simulink model "ErskineMultiDroneFormation_5drones"  (R2019b)
settings: Solver=FixedStepAuto  StartTime=0.0  StopTime=Tsim  FixedStep=sim_dt  RelTol=1e-3
values from neighbouring files (symbols this model uses):
  controller_rate = 50    [MultiQuadInit.m]
  drone_params = setDefaultDroneParams(nDrones)    [MultiQuadInit.m]
  dt_p = 0.2    [MultiQuadInit.m]    (also in setSimConditions.m)
  edges = [1,2 ... (first row only)    [MultiQuadInit.m]    (also in setSimConditions.m)
  g = 9.81    [MultiQuadInit.m]
  N_p = 5    [MultiQuadInit.m]    (also in setSimConditions.m)
  nDrones = 3    [MultiQuadInit.m]
  omega0 = zeros(3,nDrones)    [MultiQuadInit.m]    (also in setSimConditions.m)
  p0 = scale*(rand(3,nDrones) - [0.5;0.5;0])    [MultiQuadInit.m]    (also in setSimConditions.m = scale*(rand(3,nDrones) - [1/2;1/2;0]))
  q0 = zeros(4,nDrones); q0(1,:) = ones(1,nDrones)    [MultiQuadInit.m]    (also in setSimConditions.m)
  sim_dt = 0.005    [MultiQuadInit.m]
  v0 = zeros(3, nDrones)    [MultiQuadInit.m]    (also in setSimConditions.m)
undefined symbols (not defined in the file or in its folder): camera_noise
libraries: vrlib x13
(part 1 of 4)
settings Model: Creator=julian  LastModifiedBy=julian

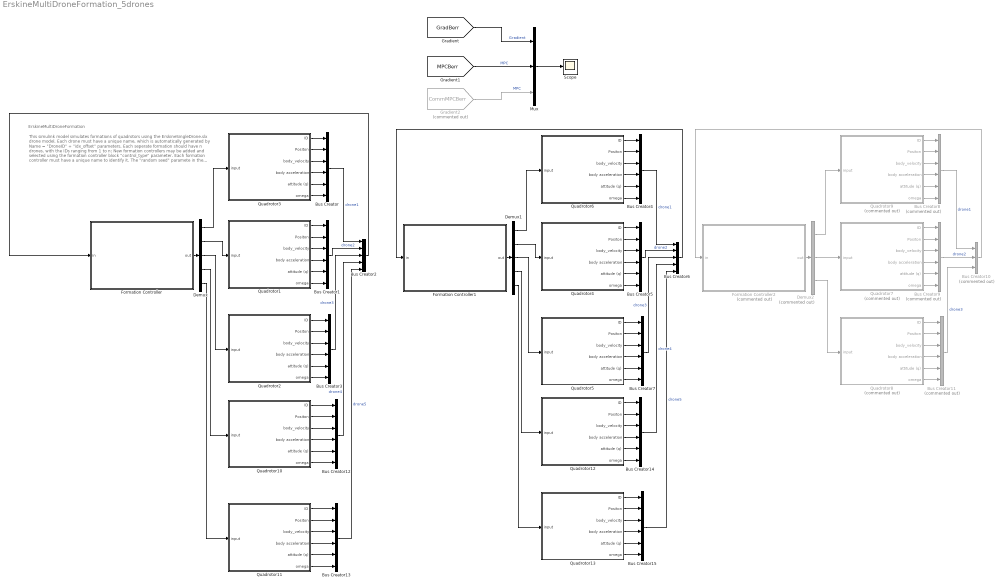
== system ErskineMultiDroneFormation_5drones ==
  note: This simulink model simulates formations of quadrotors using the
      | ErskineSingleDrone.slx drone model.  Each drone must have a unique name,
      | which is automatically generated by Name = "DroneID" + "idx_offset" parameters.
      | Each seperate formation should have n drones, with the IDs ranging from 1 to n;
      |
      | New formation controllers may be added and selected using the formation
      | controller block "control_type" parameter. Each formation controller must have a
      | unique name to identify it. The "random seed" paramete in the formation control block sets the random noise seed for the controller measurements.
      |
      | Initial conditions, parameters, and the FormationStateBus must be generated for n drones (see initialization script)
  note: ErskineMultiDroneFormation
  "  Quadrotor1" : Subsystem  mask{control_type_param=2: Body Velocity + Yawrate, DroneID=2, DroneName=Drone2, idx_offset=0}
      mask prompts: control_type_param "Controller type"; DroneName "Drone Name"; idx_offset "Index Offset"
      mask TypeOptions control_type_param: 1: Position + Yaw | 2: Body Velocity + Yawrate | 3: Body Acceleration + Yawrate | 4: Thrust + Attitude | 5: Thrust + Body Rate | 6: Body Wrench
      mask TypeOptions DroneID: 1 | 2 | 3 | 4 | 5 | 6 | 7 | 8 | 9
      mask Callback DroneID:
      | ID = get_param(gcb,'DroneID');
      | offset = get_param(gcb,'idx_offset');
      | if ischar(ID)
      |   ID = str2num(ID);
      | end
      | if ischar(offset)
      |   offset = str2num(offset);
      | end
      | nameID = ID + offset;
      | set_param(gcb,'DroneName',["Drone"+num2str(nameID)]);
      mask Callback DroneName: set_param([gcb,'/To Workspace'],'VariableName',[get_param(gcb,'DroneName')]);
      mask Callback idx_offset:
      | ID = get_param(gcb,'DroneID');
      | offset = get_param(gcb,'idx_offset');
      | if ischar(ID)
      |   ID = str2num(ID);
      | end
      | if ischar(offset)
      |   offset = str2num(offset);
      | end
      | nameID = ID + offset;
      | set_param(gcb,'DroneName',["Drone"+num2str(nameID)]);
      mask DialogControl Control4 Prompt: click to choose controller
      mask Display:
      | image('Format/drone_image.png'); % Use "Edit Image" on toolstrip to change.
      | Name = get_param(gcb,'DroneName');
      | ID = get_param(gcb,'DroneID');
      | C_mode = get_param(gcb,'control_type_param');
      | C_mode(1:2) = [];
      | color('red')
      | ID = "ID = "+ID;
      | color('red')
      | text(0.5, 0.25, Name, 'horizontalAlignment', 'center')
      | color('red')
      | text(0.5, 0.15, ID, 'horizontalAlignment', 'center')
      | color('blue');
      | text(0.5, 0.05, C_mode, 'horizontalAlignment', 'center')
  "  Quadrotor10" : Subsystem  mask{control_type_param=2: Body Velocity + Yawrate, DroneID=4, DroneName=Drone4, idx_offset=0}
      mask prompts: control_type_param "Controller type"; DroneName "Drone Name"; idx_offset "Index Offset"
      mask TypeOptions control_type_param: 1: Position + Yaw | 2: Body Velocity + Yawrate | 3: Body Acceleration + Yawrate | 4: Thrust + Attitude | 5: Thrust + Body Rate | 6: Body Wrench
      mask TypeOptions DroneID: 1 | 2 | 3 | 4 | 5 | 6 | 7 | 8 | 9
      mask Callback DroneID:
      | ID = get_param(gcb,'DroneID');
      | offset = get_param(gcb,'idx_offset');
      | if ischar(ID)
      |   ID = str2num(ID);
      | end
      | if ischar(offset)
      |   offset = str2num(offset);
      | end
      | nameID = ID + offset;
      | set_param(gcb,'DroneName',["Drone"+num2str(nameID)]);
      mask Callback DroneName: set_param([gcb,'/To Workspace'],'VariableName',[get_param(gcb,'DroneName')]);
      mask Callback idx_offset:
      | ID = get_param(gcb,'DroneID');
      | offset = get_param(gcb,'idx_offset');
      | if ischar(ID)
      |   ID = str2num(ID);
      | end
      | if ischar(offset)
      |   offset = str2num(offset);
      | end
      | nameID = ID + offset;
      | set_param(gcb,'DroneName',["Drone"+num2str(nameID)]);
      mask DialogControl Control4 Prompt: click to choose controller
      mask Display:
      | image('Format/drone_image.png'); % Use "Edit Image" on toolstrip to change.
      | Name = get_param(gcb,'DroneName');
      | ID = get_param(gcb,'DroneID');
      | C_mode = get_param(gcb,'control_type_param');
      | C_mode(1:2) = [];
      | color('red')
      | ID = "ID = "+ID;
      | color('red')
      | text(0.5, 0.25, Name, 'horizontalAlignment', 'center')
      | color('red')
      | text(0.5, 0.15, ID, 'horizontalAlignment', 'center')
      | color('blue');
      | text(0.5, 0.05, C_mode, 'horizontalAlignment', 'center')
  "  Quadrotor11" : Subsystem  mask{control_type_param=2: Body Velocity + Yawrate, DroneID=5, DroneName=Drone5, idx_offset=0}
      mask prompts: control_type_param "Controller type"; DroneName "Drone Name"; idx_offset "Index Offset"
      mask TypeOptions control_type_param: 1: Position + Yaw | 2: Body Velocity + Yawrate | 3: Body Acceleration + Yawrate | 4: Thrust + Attitude | 5: Thrust + Body Rate | 6: Body Wrench
      mask TypeOptions DroneID: 1 | 2 | 3 | 4 | 5 | 6 | 7 | 8 | 9
      mask Callback DroneID:
      | ID = get_param(gcb,'DroneID');
      | offset = get_param(gcb,'idx_offset');
      | if ischar(ID)
      |   ID = str2num(ID);
      | end
      | if ischar(offset)
      |   offset = str2num(offset);
      | end
      | nameID = ID + offset;
      | set_param(gcb,'DroneName',["Drone"+num2str(nameID)]);
      mask Callback DroneName: set_param([gcb,'/To Workspace'],'VariableName',[get_param(gcb,'DroneName')]);
      mask Callback idx_offset:
      | ID = get_param(gcb,'DroneID');
      | offset = get_param(gcb,'idx_offset');
      | if ischar(ID)
      |   ID = str2num(ID);
      | end
      | if ischar(offset)
      |   offset = str2num(offset);
      | end
      | nameID = ID + offset;
      | set_param(gcb,'DroneName',["Drone"+num2str(nameID)]);
      mask DialogControl Control4 Prompt: click to choose controller
      mask Display:
      | image('Format/drone_image.png'); % Use "Edit Image" on toolstrip to change.
      | Name = get_param(gcb,'DroneName');
      | ID = get_param(gcb,'DroneID');
      | C_mode = get_param(gcb,'control_type_param');
      | C_mode(1:2) = [];
      | color('red')
      | ID = "ID = "+ID;
      | color('red')
      | text(0.5, 0.25, Name, 'horizontalAlignment', 'center')
      | color('red')
      | text(0.5, 0.15, ID, 'horizontalAlignment', 'center')
      | color('blue');
      | text(0.5, 0.05, C_mode, 'horizontalAlignment', 'center')
  "  Quadrotor12" : Subsystem  mask{control_type_param=5: Thrust + Body Rate, DroneID=4, DroneName=Drone9, idx_offset=5}
      mask prompts: control_type_param "Controller type"; DroneName "Drone Name"; idx_offset "Index Offset"
      mask TypeOptions control_type_param: 1: Position + Yaw | 2: Body Velocity + Yawrate | 3: Body Acceleration + Yawrate | 4: Thrust + Attitude | 5: Thrust + Body Rate | 6: Body Wrench
      mask TypeOptions DroneID: 1 | 2 | 3 | 4 | 5 | 6 | 7 | 8 | 9
      mask Callback DroneID:
      | ID = get_param(gcb,'DroneID');
      | offset = get_param(gcb,'idx_offset');
      | if ischar(ID)
      |   ID = str2num(ID);
      | end
      | if ischar(offset)
      |   offset = str2num(offset);
      | end
      | nameID = ID + offset;
      | set_param(gcb,'DroneName',["Drone"+num2str(nameID)]);
      mask Callback DroneName: set_param([gcb,'/To Workspace'],'VariableName',[get_param(gcb,'DroneName')]);
      mask Callback idx_offset:
      | ID = get_param(gcb,'DroneID');
      | offset = get_param(gcb,'idx_offset');
      | if ischar(ID)
      |   ID = str2num(ID);
      | end
      | if ischar(offset)
      |   offset = str2num(offset);
      | end
      | nameID = ID + offset;
      | set_param(gcb,'DroneName',["Drone"+num2str(nameID)]);
      mask DialogControl Control4 Prompt: click to choose controller
      mask Display:
      | image('Format/drone_image.png'); % Use "Edit Image" on toolstrip to change.
      | Name = get_param(gcb,'DroneName');
      | ID = get_param(gcb,'DroneID');
      | C_mode = get_param(gcb,'control_type_param');
      | C_mode(1:2) = [];
      | color('red')
      | ID = "ID = "+ID;
      | color('red')
      | text(0.5, 0.25, Name, 'horizontalAlignment', 'center')
      | color('red')
      | text(0.5, 0.15, ID, 'horizontalAlignment', 'center')
      | color('blue');
      | text(0.5, 0.05, C_mode, 'horizontalAlignment', 'center')
  "  Quadrotor13" : Subsystem  mask{control_type_param=5: Thrust + Body Rate, DroneID=5, DroneName=Drone10, idx_offset=5}
      mask prompts: control_type_param "Controller type"; DroneName "Drone Name"; idx_offset "Index Offset"
      mask TypeOptions control_type_param: 1: Position + Yaw | 2: Body Velocity + Yawrate | 3: Body Acceleration + Yawrate | 4: Thrust + Attitude | 5: Thrust + Body Rate | 6: Body Wrench
      mask TypeOptions DroneID: 1 | 2 | 3 | 4 | 5 | 6 | 7 | 8 | 9
      mask Callback DroneID:
      | ID = get_param(gcb,'DroneID');
      | offset = get_param(gcb,'idx_offset');
      | if ischar(ID)
      |   ID = str2num(ID);
      | end
      | if ischar(offset)
      |   offset = str2num(offset);
      | end
      | nameID = ID + offset;
      | set_param(gcb,'DroneName',["Drone"+num2str(nameID)]);
      mask Callback DroneName: set_param([gcb,'/To Workspace'],'VariableName',[get_param(gcb,'DroneName')]);
      mask Callback idx_offset:
      | ID = get_param(gcb,'DroneID');
      | offset = get_param(gcb,'idx_offset');
      | if ischar(ID)
      |   ID = str2num(ID);
      | end
      | if ischar(offset)
      |   offset = str2num(offset);
      | end
      | nameID = ID + offset;
      | set_param(gcb,'DroneName',["Drone"+num2str(nameID)]);
      mask DialogControl Control4 Prompt: click to choose controller
      mask Display:
      | image('Format/drone_image.png'); % Use "Edit Image" on toolstrip to change.
      | Name = get_param(gcb,'DroneName');
      | ID = get_param(gcb,'DroneID');
      | C_mode = get_param(gcb,'control_type_param');
      | C_mode(1:2) = [];
      | color('red')
      | ID = "ID = "+ID;
      | color('red')
      | text(0.5, 0.25, Name, 'horizontalAlignment', 'center')
      | color('red')
      | text(0.5, 0.15, ID, 'horizontalAlignment', 'center')
      | color('blue');
      | text(0.5, 0.05, C_mode, 'horizontalAlignment', 'center')
  "  Quadrotor2" : Subsystem  mask{control_type_param=2: Body Velocity + Yawrate, DroneID=3, DroneName=Drone3, idx_offset=0}
      mask prompts: control_type_param "Controller type"; DroneName "Drone Name"; idx_offset "Index Offset"
      mask TypeOptions control_type_param: 1: Position + Yaw | 2: Body Velocity + Yawrate | 3: Body Acceleration + Yawrate | 4: Thrust + Attitude | 5: Thrust + Body Rate | 6: Body Wrench
      mask TypeOptions DroneID: 1 | 2 | 3 | 4 | 5 | 6 | 7 | 8 | 9
      mask Callback DroneID:
      | ID = get_param(gcb,'DroneID');
      | offset = get_param(gcb,'idx_offset');
      | if ischar(ID)
      |   ID = str2num(ID);
      | end
      | if ischar(offset)
      |   offset = str2num(offset);
      | end
      | nameID = ID + offset;
      | set_param(gcb,'DroneName',["Drone"+num2str(nameID)]);
      mask Callback DroneName: set_param([gcb,'/To Workspace'],'VariableName',[get_param(gcb,'DroneName')]);
      mask Callback idx_offset:
      | ID = get_param(gcb,'DroneID');
      | offset = get_param(gcb,'idx_offset');
      | if ischar(ID)
      |   ID = str2num(ID);
      | end
      | if ischar(offset)
      |   offset = str2num(offset);
      | end
      | nameID = ID + offset;
      | set_param(gcb,'DroneName',["Drone"+num2str(nameID)]);
      mask DialogControl Control4 Prompt: click to choose controller
      mask Display:
      | image('Format/drone_image.png'); % Use "Edit Image" on toolstrip to change.
      | Name = get_param(gcb,'DroneName');
      | ID = get_param(gcb,'DroneID');
      | C_mode = get_param(gcb,'control_type_param');
      | C_mode(1:2) = [];
      | color('red')
      | ID = "ID = "+ID;
      | color('red')
      | text(0.5, 0.25, Name, 'horizontalAlignment', 'center')
      | color('red')
      | text(0.5, 0.15, ID, 'horizontalAlignment', 'center')
      | color('blue');
      | text(0.5, 0.05, C_mode, 'horizontalAlignment', 'center')
  "  Quadrotor3" : Subsystem  mask{control_type_param=2: Body Velocity + Yawrate, DroneID=1, DroneName=Drone1, idx_offset=0}
      mask prompts: control_type_param "Controller type"; DroneName "Drone Name"; idx_offset "Index Offset"
      mask TypeOptions control_type_param: 1: Position + Yaw | 2: Body Velocity + Yawrate | 3: Body Acceleration + Yawrate | 4: Thrust + Attitude | 5: Thrust + Body Rate | 6: Body Wrench
      mask TypeOptions DroneID: 1 | 2 | 3 | 4 | 5 | 6 | 7 | 8 | 9
      mask Callback DroneID:
      | ID = get_param(gcb,'DroneID');
      | offset = get_param(gcb,'idx_offset');
      | if ischar(ID)
      |   ID = str2num(ID);
      | end
      | if ischar(offset)
      |   offset = str2num(offset);
      | end
      | nameID = ID + offset;
      | set_param(gcb,'DroneName',["Drone"+num2str(nameID)]);
      mask Callback DroneName: set_param([gcb,'/To Workspace'],'VariableName',[get_param(gcb,'DroneName')]);
      mask Callback idx_offset:
      | ID = get_param(gcb,'DroneID');
      | offset = get_param(gcb,'idx_offset');
      | if ischar(ID)
      |   ID = str2num(ID);
      | end
      | if ischar(offset)
      |   offset = str2num(offset);
      | end
      | nameID = ID + offset;
      | set_param(gcb,'DroneName',["Drone"+num2str(nameID)]);
      mask DialogControl Control4 Prompt: click to choose controller
      mask Display:
      | image('Format/drone_image.png'); % Use "Edit Image" on toolstrip to change.
      | Name = get_param(gcb,'DroneName');
      | ID = get_param(gcb,'DroneID');
      | C_mode = get_param(gcb,'control_type_param');
      | C_mode(1:2) = [];
      | color('red')
      | ID = "ID = "+ID;
      | color('red')
      | text(0.5, 0.25, Name, 'horizontalAlignment', 'center')
      | color('red')
      | text(0.5, 0.15, ID, 'horizontalAlignment', 'center')
      | color('blue');
      | text(0.5, 0.05, C_mode, 'horizontalAlignment', 'center')
  "  Quadrotor4" : Subsystem  mask{control_type_param=5: Thrust + Body Rate, DroneID=2, DroneName=Drone7, idx_offset=5}
      mask prompts: control_type_param "Controller type"; DroneName "Drone Name"; idx_offset "Index Offset"
      mask TypeOptions control_type_param: 1: Position + Yaw | 2: Body Velocity + Yawrate | 3: Body Acceleration + Yawrate | 4: Thrust + Attitude | 5: Thrust + Body Rate | 6: Body Wrench
      mask TypeOptions DroneID: 1 | 2 | 3 | 4 | 5 | 6 | 7 | 8 | 9
      mask Callback DroneID:
      | ID = get_param(gcb,'DroneID');
      | offset = get_param(gcb,'idx_offset');
      | if ischar(ID)
      |   ID = str2num(ID);
      | end
      | if ischar(offset)
      |   offset = str2num(offset);
      | end
      | nameID = ID + offset;
      | set_param(gcb,'DroneName',["Drone"+num2str(nameID)]);
      mask Callback DroneName: set_param([gcb,'/To Workspace'],'VariableName',[get_param(gcb,'DroneName')]);
      mask Callback idx_offset:
      | ID = get_param(gcb,'DroneID');
      | offset = get_param(gcb,'idx_offset');
      | if ischar(ID)
      |   ID = str2num(ID);
      | end
      | if ischar(offset)
      |   offset = str2num(offset);
      | end
      | nameID = ID + offset;
      | set_param(gcb,'DroneName',["Drone"+num2str(nameID)]);
      mask DialogControl Control4 Prompt: click to choose controller
      mask Display:
      | image('Format/drone_image.png'); % Use "Edit Image" on toolstrip to change.
      | Name = get_param(gcb,'DroneName');
      | ID = get_param(gcb,'DroneID');
      | C_mode = get_param(gcb,'control_type_param');
      | C_mode(1:2) = [];
      | color('red')
      | ID = "ID = "+ID;
      | color('red')
      | text(0.5, 0.25, Name, 'horizontalAlignment', 'center')
      | color('red')
      | text(0.5, 0.15, ID, 'horizontalAlignment', 'center')
      | color('blue');
      | text(0.5, 0.05, C_mode, 'horizontalAlignment', 'center')
  "  Quadrotor5" : Subsystem  mask{control_type_param=5: Thrust + Body Rate, DroneID=3, DroneName=Drone8, idx_offset=5}
      mask prompts: control_type_param "Controller type"; DroneName "Drone Name"; idx_offset "Index Offset"
      mask TypeOptions control_type_param: 1: Position + Yaw | 2: Body Velocity + Yawrate | 3: Body Acceleration + Yawrate | 4: Thrust + Attitude | 5: Thrust + Body Rate | 6: Body Wrench
      mask TypeOptions DroneID: 1 | 2 | 3 | 4 | 5 | 6 | 7 | 8 | 9
      mask Callback DroneID:
      | ID = get_param(gcb,'DroneID');
      | offset = get_param(gcb,'idx_offset');
      | if ischar(ID)
      |   ID = str2num(ID);
      | end
      | if ischar(offset)
      |   offset = str2num(offset);
      | end
      | nameID = ID + offset;
      | set_param(gcb,'DroneName',["Drone"+num2str(nameID)]);
      mask Callback DroneName: set_param([gcb,'/To Workspace'],'VariableName',[get_param(gcb,'DroneName')]);
      mask Callback idx_offset:
      | ID = get_param(gcb,'DroneID');
      | offset = get_param(gcb,'idx_offset');
      | if ischar(ID)
      |   ID = str2num(ID);
      | end
      | if ischar(offset)
      |   offset = str2num(offset);
      | end
      | nameID = ID + offset;
      | set_param(gcb,'DroneName',["Drone"+num2str(nameID)]);
      mask DialogControl Control4 Prompt: click to choose controller
      mask Display:
      | image('Format/drone_image.png'); % Use "Edit Image" on toolstrip to change.
      | Name = get_param(gcb,'DroneName');
      | ID = get_param(gcb,'DroneID');
      | C_mode = get_param(gcb,'control_type_param');
      | C_mode(1:2) = [];
      | color('red')
      | ID = "ID = "+ID;
      | color('red')
      | text(0.5, 0.25, Name, 'horizontalAlignment', 'center')
      | color('red')
      | text(0.5, 0.15, ID, 'horizontalAlignment', 'center')
      | color('blue');
      | text(0.5, 0.05, C_mode, 'horizontalAlignment', 'center')
  "  Quadrotor6" : Subsystem  mask{control_type_param=5: Thrust + Body Rate, DroneID=1, DroneName=Drone6, idx_offset=5}
      mask prompts: control_type_param "Controller type"; DroneName "Drone Name"; idx_offset "Index Offset"
      mask TypeOptions control_type_param: 1: Position + Yaw | 2: Body Velocity + Yawrate | 3: Body Acceleration + Yawrate | 4: Thrust + Attitude | 5: Thrust + Body Rate | 6: Body Wrench
      mask TypeOptions DroneID: 1 | 2 | 3 | 4 | 5 | 6 | 7 | 8 | 9
      mask Callback DroneID:
      | ID = get_param(gcb,'DroneID');
      | offset = get_param(gcb,'idx_offset');
      | if ischar(ID)
      |   ID = str2num(ID);
      | end
      | if ischar(offset)
      |   offset = str2num(offset);
      | end
      | nameID = ID + offset;
      | set_param(gcb,'DroneName',["Drone"+num2str(nameID)]);
      mask Callback DroneName: set_param([gcb,'/To Workspace'],'VariableName',[get_param(gcb,'DroneName')]);
      mask Callback idx_offset:
      | ID = get_param(gcb,'DroneID');
      | offset = get_param(gcb,'idx_offset');
      | if ischar(ID)
      |   ID = str2num(ID);
      | end
      | if ischar(offset)
      |   offset = str2num(offset);
      | end
      | nameID = ID + offset;
      | set_param(gcb,'DroneName',["Drone"+num2str(nameID)]);
      mask DialogControl Control4 Prompt: click to choose controller
      mask Display:
      | image('Format/drone_image.png'); % Use "Edit Image" on toolstrip to change.
      | Name = get_param(gcb,'DroneName');
      | ID = get_param(gcb,'DroneID');
      | C_mode = get_param(gcb,'control_type_param');
      | C_mode(1:2) = [];
      | color('red')
      | ID = "ID = "+ID;
      | color('red')
      | text(0.5, 0.25, Name, 'horizontalAlignment', 'center')
      | color('red')
      | text(0.5, 0.15, ID, 'horizontalAlignment', 'center')
      | color('blue');
      | text(0.5, 0.05, C_mode, 'horizontalAlignment', 'center')
  "  Quadrotor7" : Subsystem  Commented=on  mask{control_type_param=5: Thrust + Body Rate, DroneID=2, DroneName=Drone8, idx_offset=6}
      mask prompts: control_type_param "Controller type"; DroneName "Drone Name"; idx_offset "Index Offset"
      mask TypeOptions control_type_param: 1: Position + Yaw | 2: Body Velocity + Yawrate | 3: Body Acceleration + Yawrate | 4: Thrust + Attitude | 5: Thrust + Body Rate | 6: Body Wrench
      mask TypeOptions DroneID: 1 | 2 | 3 | 4 | 5 | 6 | 7 | 8 | 9
      mask Callback DroneID:
      | ID = get_param(gcb,'DroneID');
      | offset = get_param(gcb,'idx_offset');
      | if ischar(ID)
      |   ID = str2num(ID);
      | end
      | if ischar(offset)
      |   offset = str2num(offset);
      | end
      | nameID = ID + offset;
      | set_param(gcb,'DroneName',["Drone"+num2str(nameID)]);
      mask Callback DroneName: set_param([gcb,'/To Workspace'],'VariableName',[get_param(gcb,'DroneName')]);
      mask Callback idx_offset:
      | ID = get_param(gcb,'DroneID');
      | offset = get_param(gcb,'idx_offset');
      | if ischar(ID)
      |   ID = str2num(ID);
      | end
      | if ischar(offset)
      |   offset = str2num(offset);
      | end
      | nameID = ID + offset;
      | set_param(gcb,'DroneName',["Drone"+num2str(nameID)]);
      mask DialogControl Control4 Prompt: click to choose controller
      mask Display:
      | image('Format/drone_image.png'); % Use "Edit Image" on toolstrip to change.
      | Name = get_param(gcb,'DroneName');
      | ID = get_param(gcb,'DroneID');
      | C_mode = get_param(gcb,'control_type_param');
      | C_mode(1:2) = [];
      | color('red')
      | ID = "ID = "+ID;
      | color('red')
      | text(0.5, 0.25, Name, 'horizontalAlignment', 'center')
      | color('red')
      | text(0.5, 0.15, ID, 'horizontalAlignment', 'center')
      | color('blue');
      | text(0.5, 0.05, C_mode, 'horizontalAlignment', 'center')
  "  Quadrotor8" : Subsystem  Commented=on  mask{control_type_param=5: Thrust + Body Rate, DroneID=3, DroneName=Drone9, idx_offset=6}
      mask prompts: control_type_param "Controller type"; DroneName "Drone Name"; idx_offset "Index Offset"
      mask TypeOptions control_type_param: 1: Position + Yaw | 2: Body Velocity + Yawrate | 3: Body Acceleration + Yawrate | 4: Thrust + Attitude | 5: Thrust + Body Rate | 6: Body Wrench
      mask TypeOptions DroneID: 1 | 2 | 3 | 4 | 5 | 6 | 7 | 8 | 9
      mask Callback DroneID:
      | ID = get_param(gcb,'DroneID');
      | offset = get_param(gcb,'idx_offset');
      | if ischar(ID)
      |   ID = str2num(ID);
      | end
      | if ischar(offset)
      |   offset = str2num(offset);
      | end
      | nameID = ID + offset;
      | set_param(gcb,'DroneName',["Drone"+num2str(nameID)]);
      mask Callback DroneName: set_param([gcb,'/To Workspace'],'VariableName',[get_param(gcb,'DroneName')]);
      mask Callback idx_offset:
      | ID = get_param(gcb,'DroneID');
      | offset = get_param(gcb,'idx_offset');
      | if ischar(ID)
      |   ID = str2num(ID);
      | end
      | if ischar(offset)
      |   offset = str2num(offset);
      | end
      | nameID = ID + offset;
      | set_param(gcb,'DroneName',["Drone"+num2str(nameID)]);
      mask DialogControl Control4 Prompt: click to choose controller
      mask Display:
      | image('Format/drone_image.png'); % Use "Edit Image" on toolstrip to change.
      | Name = get_param(gcb,'DroneName');
      | ID = get_param(gcb,'DroneID');
      | C_mode = get_param(gcb,'control_type_param');
      | C_mode(1:2) = [];
      | color('red')
      | ID = "ID = "+ID;
      | color('red')
      | text(0.5, 0.25, Name, 'horizontalAlignment', 'center')
      | color('red')
      | text(0.5, 0.15, ID, 'horizontalAlignment', 'center')
      | color('blue');
      | text(0.5, 0.05, C_mode, 'horizontalAlignment', 'center')
  "  Quadrotor9" : Subsystem  Commented=on  mask{control_type_param=5: Thrust + Body Rate, DroneID=1, DroneName=Drone7, idx_offset=6}
      mask prompts: control_type_param "Controller type"; DroneName "Drone Name"; idx_offset "Index Offset"
      mask TypeOptions control_type_param: 1: Position + Yaw | 2: Body Velocity + Yawrate | 3: Body Acceleration + Yawrate | 4: Thrust + Attitude | 5: Thrust + Body Rate | 6: Body Wrench
      mask TypeOptions DroneID: 1 | 2 | 3 | 4 | 5 | 6 | 7 | 8 | 9
      mask Callback DroneID:
      | ID = get_param(gcb,'DroneID');
      | offset = get_param(gcb,'idx_offset');
      | if ischar(ID)
      |   ID = str2num(ID);
      | end
      | if ischar(offset)
      |   offset = str2num(offset);
      | end
      | nameID = ID + offset;
      | set_param(gcb,'DroneName',["Drone"+num2str(nameID)]);
      mask Callback DroneName: set_param([gcb,'/To Workspace'],'VariableName',[get_param(gcb,'DroneName')]);
      mask Callback idx_offset:
      | ID = get_param(gcb,'DroneID');
      | offset = get_param(gcb,'idx_offset');
      | if ischar(ID)
      |   ID = str2num(ID);
      | end
      | if ischar(offset)
      |   offset = str2num(offset);
      | end
      | nameID = ID + offset;
      | set_param(gcb,'DroneName',["Drone"+num2str(nameID)]);
      mask DialogControl Control4 Prompt: click to choose controller
      mask Display:
      | image('Format/drone_image.png'); % Use "Edit Image" on toolstrip to change.
      | Name = get_param(gcb,'DroneName');
      | ID = get_param(gcb,'DroneID');
      | C_mode = get_param(gcb,'control_type_param');
      | C_mode(1:2) = [];
      | color('red')
      | ID = "ID = "+ID;
      | color('red')
      | text(0.5, 0.25, Name, 'horizontalAlignment', 'center')
      | color('red')
      | text(0.5, 0.15, ID, 'horizontalAlignment', 'center')
      | color('blue');
      | text(0.5, 0.05, C_mode, 'horizontalAlignment', 'center')
  Bus Creator{,1,3..5,7,12..15} (10 alike) : BusCreator  Inputs=6  OutDataTypeStr=Bus: DroneStateBus
      settings: InheritFromInputs=off
  Bus Creator10 : BusCreator  Commented=on  Inputs=3  OutDataTypeStr=Bus: FormationStateBus  NonVirtualBus=on
      settings: InheritFromInputs=off
  Bus Creator11 : BusCreator  Commented=on  Inputs=6  OutDataTypeStr=Bus: DroneStateBus
      settings: InheritFromInputs=off
  Bus Creator2 : BusCreator  Inputs=5  OutDataTypeStr=Bus: FormationStateBus  NonVirtualBus=on
      settings: InheritFromInputs=off
  Bus Creator6 : BusCreator  Inputs=5  OutDataTypeStr=Bus: FormationStateBus  NonVirtualBus=on
      settings: InheritFromInputs=off
  Bus Creator8 : BusCreator  Commented=on  Inputs=6  OutDataTypeStr=Bus: DroneStateBus
      settings: InheritFromInputs=off
  Bus Creator9 : BusCreator  Commented=on  Inputs=6  OutDataTypeStr=Bus: DroneStateBus
      settings: InheritFromInputs=off
  Demux : Demux  Outputs=5
  Demux1 : Demux  Outputs=5
  Demux2 : Demux  Commented=on  Outputs=3
  Formation Controller : Subsystem  mask(FormationController){seed_type=Custom, rng_seed=1, control_type=1: Gradient, out_name=Gradient}
      mask prompts: seed_type "Random Seed"; rng_seed "Custom Seed"; control_type "Formation Control Type"; out_name "Out Name"
      mask TypeOptions seed_type: Random | Custom
      mask Callback seed_type:
      | box_A = get_param(gcb, 'seed_type');
      | m = Simulink.Mask.get(gcb);
      | box_B = m.getParameter('rng_seed');
      | 
      | if strcmp(box_A, 'Random')
      |     seed = randi([1,10000]);
      |     set_param(gcb,'rng_seed', num2str(seed));
      |     box_B.Enabled = 'off';
      | else
      |     box_B.Enabled = 'on';
      | end
      mask TypeOptions control_type: 1: Gradient | 2: Basic MPC | 3: Communicating MPC
      mask Callback out_name: set_param([gcb,'/To Workspace'],'VariableName',[get_param(gcb,'out_name')]);
      mask Display:
      | image('$imagefile'); % Use "Edit Image" on toolstrip to change.
      | type = get_param(gcb,'control_type');
      | color('red')
      | text(0.5, 0.25, type, 'horizontalAlignment', 'center')
  Formation Controller1 : Subsystem  mask(FormationController){seed_type=Custom, rng_seed=1, control_type=2: Basic MPC, out_name=SimpleMPC}
      mask prompts: seed_type "Random Seed"; rng_seed "Custom Seed"; control_type "Formation Control Type"; out_name "Out Name"
      mask TypeOptions seed_type: Random | Custom
      mask Callback seed_type:
      | box_A = get_param(gcb, 'seed_type');
      | m = Simulink.Mask.get(gcb);
      | box_B = m.getParameter('rng_seed');
      | 
      | if strcmp(box_A, 'Random')
      |     seed = randi([1,10000]);
      |     set_param(gcb,'rng_seed', num2str(seed));
      |     box_B.Enabled = 'off';
      | else
      |     box_B.Enabled = 'on';
      | end
      mask TypeOptions control_type: 1: Gradient | 2: Basic MPC | 3: Communicating MPC
      mask Callback out_name: set_param([gcb,'/To Workspace'],'VariableName',[get_param(gcb,'out_name')]);
      mask Display:
      | image('$imagefile'); % Use "Edit Image" on toolstrip to change.
      | type = get_param(gcb,'control_type');
      | color('red');
      | text(0.5, 0.25, type, 'horizontalAlignment', 'center');
  Formation Controller2 : Subsystem  Commented=on  mask(FormationController){seed_type=Random, rng_seed=1712, control_type=3: Communicating MPC, out_name=CommunicatingMPC}
      mask prompts: seed_type "Random Seed"; rng_seed "Custom Seed"; control_type "Formation Control Type"; out_name "Out Name"
      mask TypeOptions seed_type: Random | Custom
      mask Callback seed_type:
      | box_A = get_param(gcb, 'seed_type');
      | m = Simulink.Mask.get(gcb);
      | box_B = m.getParameter('rng_seed');
      | 
      | if strcmp(box_A, 'Random')
      |     seed = randi([1,10000]);
      |     set_param(gcb,'rng_seed', num2str(seed));
      |     box_B.Enabled = 'off';
      | else
      |     box_B.Enabled = 'on';
      | end
      mask TypeOptions control_type: 1: Gradient | 2: Basic MPC | 3: Communicating MPC
      mask Callback out_name: set_param([gcb,'/To Workspace'],'VariableName',[get_param(gcb,'out_name')]);
      mask Display:
      | image('$imagefile'); % Use "Edit Image" on toolstrip to change.
      | type = get_param(gcb,'control_type');
      | color('red')
      | text(0.5, 0.25, type, 'horizontalAlignment', 'center')
  Gradient2 : From  Commented=on  GotoTag=CommMPCBerr  TagVisibility=global
  Mux : Mux  Inputs=3
  Scope : Scope
  wires:
  "  Quadrotor3"/6(omega) -> Bus Creator/6
  "  Quadrotor3"/5(attitude (q)) -> Bus Creator/5
  "  Quadrotor3"/4(body acceleration) -> Bus Creator/4
  "  Quadrotor3"/3(body_velocity) -> Bus Creator/3
  "  Quadrotor3"/2(Positon) -> Bus Creator/2
  "  Quadrotor3"/1(ID) -> Bus Creator/1
  "  Quadrotor1"/1(ID) -> Bus Creator1/1
  "  Quadrotor1"/2(Positon) -> Bus Creator1/2
  "  Quadrotor1"/3(body_velocity) -> Bus Creator1/3
  "  Quadrotor1"/4(body acceleration) -> Bus Creator1/4
  "  Quadrotor1"/5(attitude (q)) -> Bus Creator1/5
  "  Quadrotor1"/6(omega) -> Bus Creator1/6
  Bus Creator/1 -> Bus Creator2/1  "drone1"
  Bus Creator1/1 -> Bus Creator2/2  "drone2"
  Bus Creator2/1 -> Formation Controller/1(in)
  Formation Controller/1(out) -> Demux/1
  "  Quadrotor2"/1(ID) -> Bus Creator3/1
  "  Quadrotor2"/2(Positon) -> Bus Creator3/2
  "  Quadrotor2"/3(body_velocity) -> Bus Creator3/3
  "  Quadrotor2"/4(body acceleration) -> Bus Creator3/4
  "  Quadrotor2"/5(attitude (q)) -> Bus Creator3/5
  "  Quadrotor2"/6(omega) -> Bus Creator3/6
  Bus Creator3/1 -> Bus Creator2/3  "drone3"
  Demux/1 -> "  Quadrotor3"/1(input)
  Demux/2 -> "  Quadrotor1"/1(input)
  Demux/3 -> "  Quadrotor2"/1(input)
  Demux1/2 -> "  Quadrotor4"/1(input)
  "  Quadrotor5"/3(body_velocity) -> Bus Creator7/3
  "  Quadrotor6"/1(ID) -> Bus Creator4/1
  "  Quadrotor6"/4(body acceleration) -> Bus Creator4/4
  "  Quadrotor4"/1(ID) -> Bus Creator5/1
  "  Quadrotor4"/2(Positon) -> Bus Creator5/2
  "  Quadrotor6"/2(Positon) -> Bus Creator4/2
  "  Quadrotor4"/3(body_velocity) -> Bus Creator5/3
  "  Quadrotor4"/4(body acceleration) -> Bus Creator5/4
  "  Quadrotor4"/5(attitude (q)) -> Bus Creator5/5
  "  Quadrotor6"/6(omega) -> Bus Creator4/6
  Bus Creator6/1 -> Formation Controller1/1(in)
  "  Quadrotor5"/4(body acceleration) -> Bus Creator7/4
  Bus Creator4/1 -> Bus Creator6/1  "drone1"
  "  Quadrotor4"/6(omega) -> Bus Creator5/6
  Bus Creator5/1 -> Bus Creator6/2  "drone2"
  "  Quadrotor5"/2(Positon) -> Bus Creator7/2
  Demux1/1 -> "  Quadrotor6"/1(input)
  Bus Creator7/1 -> Bus Creator6/3  "drone3"
  Formation Controller1/1(out) -> Demux1/1
  "  Quadrotor5"/6(omega) -> Bus Creator7/6
  "  Quadrotor6"/5(attitude (q)) -> Bus Creator4/5
  Demux1/3 -> "  Quadrotor5"/1(input)
  "  Quadrotor6"/3(body_velocity) -> Bus Creator4/3
  "  Quadrotor5"/5(attitude (q)) -> Bus Creator7/5
  "  Quadrotor5"/1(ID) -> Bus Creator7/1
  Demux2/3 -> "  Quadrotor8"/1(input)
  "  Quadrotor7"/6(omega) -> Bus Creator9/6
  "  Quadrotor9"/5(attitude (q)) -> Bus Creator8/5
  "  Quadrotor8"/3(body_velocity) -> Bus Creator11/3
  "  Quadrotor7"/5(attitude (q)) -> Bus Creator9/5
  Demux2/1 -> "  Quadrotor9"/1(input)
  "  Quadrotor8"/1(ID) -> Bus Creator11/1
  Demux2/2 -> "  Quadrotor7"/1(input)
  "  Quadrotor8"/2(Positon) -> Bus Creator11/2
  "  Quadrotor8"/4(body acceleration) -> Bus Creator11/4
  Bus Creator11/1 -> Bus Creator10/3  "drone3"
  Formation Controller2/1(out) -> Demux2/1
  "  Quadrotor7"/3(body_velocity) -> Bus Creator9/3
  "  Quadrotor9"/1(ID) -> Bus Creator8/1
  "  Quadrotor9"/4(body acceleration) -> Bus Creator8/4
  "  Quadrotor8"/6(omega) -> Bus Creator11/6
  "  Quadrotor7"/2(Positon) -> Bus Creator9/2
  Bus Creator10/1 -> Formation Controller2/1(in)
  "  Quadrotor9"/6(omega) -> Bus Creator8/6
  "  Quadrotor7"/1(ID) -> Bus Creator9/1
  Bus Creator9/1 -> Bus Creator10/2  "drone2"
  "  Quadrotor9"/2(Positon) -> Bus Creator8/2
  "  Quadrotor7"/4(body acceleration) -> Bus Creator9/4
  "  Quadrotor8"/5(attitude (q)) -> Bus Creator11/5
  Bus Creator8/1 -> Bus Creator10/1  "drone1"
  "  Quadrotor9"/3(body_velocity) -> Bus Creator8/3
  [MPCBerr] -> Mux/2  "MPC"
  [GradBerr] -> Mux/1  "Gradient"
  Mux/1 -> Scope/1
  Gradient2/1 -> Mux/3  "MPC"
  "  Quadrotor10"/6(omega) -> Bus Creator12/6
  "  Quadrotor10"/1(ID) -> Bus Creator12/1
  "  Quadrotor10"/2(Positon) -> Bus Creator12/2
  "  Quadrotor10"/4(body acceleration) -> Bus Creator12/4
  Bus Creator12/1 -> Bus Creator2/4  "drone4"
  "  Quadrotor10"/3(body_velocity) -> Bus Creator12/3
  "  Quadrotor10"/5(attitude (q)) -> Bus Creator12/5
  Demux/4 -> "  Quadrotor10"/1(input)
  "  Quadrotor11"/6(omega) -> Bus Creator13/6
  "  Quadrotor11"/1(ID) -> Bus Creator13/1
  "  Quadrotor11"/2(Positon) -> Bus Creator13/2
  "  Quadrotor11"/4(body acceleration) -> Bus Creator13/4
  Bus Creator13/1 -> Bus Creator2/5  "drone5"
  "  Quadrotor11"/3(body_velocity) -> Bus Creator13/3
  "  Quadrotor11"/5(attitude (q)) -> Bus Creator13/5
  Demux/5 -> "  Quadrotor11"/1(input)
  Bus Creator14/1 -> Bus Creator6/4  "drone4"
  "  Quadrotor13"/3(body_velocity) -> Bus Creator15/3
  "  Quadrotor12"/5(attitude (q)) -> Bus Creator14/5
  "  Quadrotor13"/5(attitude (q)) -> Bus Creator15/5
  "  Quadrotor13"/4(body acceleration) -> Bus Creator15/4
  "  Quadrotor12"/3(body_velocity) -> Bus Creator14/3
  Demux1/4 -> "  Quadrotor12"/1(input)
  "  Quadrotor13"/2(Positon) -> Bus Creator15/2
  "  Quadrotor12"/6(omega) -> Bus Creator14/6
  "  Quadrotor12"/4(body acceleration) -> Bus Creator14/4
  "  Quadrotor13"/1(ID) -> Bus Creator15/1
  "  Quadrotor13"/6(omega) -> Bus Creator15/6
  Demux1/5 -> "  Quadrotor13"/1(input)
  Bus Creator15/1 -> Bus Creator6/5  "drone5"
  "  Quadrotor12"/2(Positon) -> Bus Creator14/2
  "  Quadrotor12"/1(ID) -> Bus Creator14/1

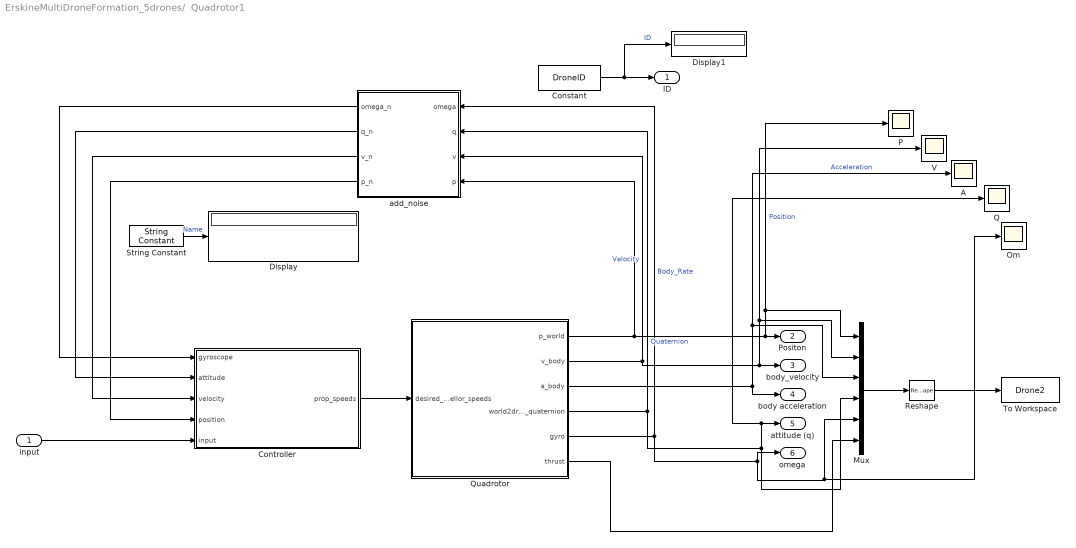
== system ErskineMultiDroneFormation_5drones/  Quadrotor1 ==
  input : Inport
  A : Scope
  Constant : Constant  Value=DroneID
  Controller : Subsystem
      mask Display: image('Format/flightController.png'); % Use "Edit Image" on toolstrip to change.
  Display : Display
  Display1 : Display
  Mux : Mux  Inputs=6
  Om : Scope
  P : Scope
  Q : Scope
  Quadrotor : Subsystem
      mask Display: image('droneHardware.jpeg'); % Use "Edit Image" on toolstrip to change.
  Reshape : Reshape
  String Constant : StringConstant  String=DroneName
  To Workspace : ToWorkspace  VariableName=Drone2  SaveFormat=Timeseries  SampleTime=-1
  V : Scope
  add_noise : MATLAB Function  TreatAsAtomicUnit=on
  ID : Outport
  Positon : Outport  Port=2
  body_velocity : Outport  Port=3
  body acceleration : Outport  Port=4
  attitude (q) : Outport  Port=5
  omega : Outport  Port=6
  wires:
  Quadrotor/5(gyro) -> Om/1, Mux/5, omega/1, add_noise/1(omega)  "Body_Rate"
  Quadrotor/1(p_world) -> add_noise/4(p), P/1, Mux/1, Positon/1  "Position"
  Quadrotor/3(a_body) -> body acceleration/1, A/1, Mux/3  "Acceleration"
  Quadrotor/4(world2drone_quaternion) -> Q/1, attitude (q)/1, Mux/4, add_noise/2(q)  "Quaternion"
  Mux/1 -> Reshape/1
  Quadrotor/2(v_body) -> V/1, Mux/2, body_velocity/1, add_noise/3(v)  "Velocity"
  Quadrotor/6(thrust) -> Mux/6
  String Constant/1 -> Display/1  "Name"
  Constant/1 -> Display1/1, ID/1  "ID"
  Reshape/1 -> To Workspace/1
  add_noise/1(omega_n) -> Controller/1(gyroscope)
  add_noise/2(q_n) -> Controller/2(attitude)
  add_noise/3(v_n) -> Controller/3(velocity)
  add_noise/4(p_n) -> Controller/4(position)
  input/1 -> Controller/5(input)
  Controller/1(prop_speeds) -> Quadrotor/1(desired_propellor_speeds)

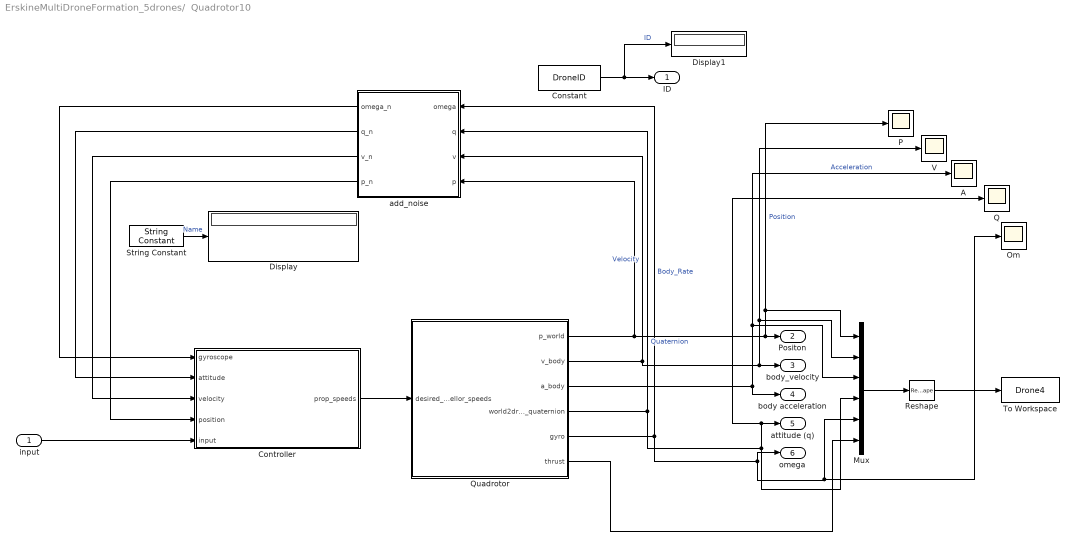
== system ErskineMultiDroneFormation_5drones/  Quadrotor10 ==
  input : Inport
  A : Scope
  Constant : Constant  Value=DroneID
  Controller : Subsystem
      mask Display: image('Format/flightController.png'); % Use "Edit Image" on toolstrip to change.
  Display : Display
  Display1 : Display
  Mux : Mux  Inputs=6
  Om : Scope
  P : Scope
  Q : Scope
  Quadrotor : Subsystem
      mask Display: image('droneHardware.jpeg'); % Use "Edit Image" on toolstrip to change.
  Reshape : Reshape
  String Constant : StringConstant  String=DroneName
  To Workspace : ToWorkspace  VariableName=Drone4  SaveFormat=Timeseries  SampleTime=-1
  V : Scope
  add_noise : MATLAB Function  TreatAsAtomicUnit=on
  ID : Outport
  Positon : Outport  Port=2
  body_velocity : Outport  Port=3
  body acceleration : Outport  Port=4
  attitude (q) : Outport  Port=5
  omega : Outport  Port=6
  wires:
  Quadrotor/5(gyro) -> Om/1, Mux/5, omega/1, add_noise/1(omega)  "Body_Rate"
  Quadrotor/1(p_world) -> add_noise/4(p), P/1, Mux/1, Positon/1  "Position"
  Quadrotor/3(a_body) -> body acceleration/1, A/1, Mux/3  "Acceleration"
  Quadrotor/4(world2drone_quaternion) -> Q/1, attitude (q)/1, Mux/4, add_noise/2(q)  "Quaternion"
  Mux/1 -> Reshape/1
  Quadrotor/2(v_body) -> V/1, Mux/2, body_velocity/1, add_noise/3(v)  "Velocity"
  Quadrotor/6(thrust) -> Mux/6
  String Constant/1 -> Display/1  "Name"
  Constant/1 -> Display1/1, ID/1  "ID"
  Reshape/1 -> To Workspace/1
  add_noise/1(omega_n) -> Controller/1(gyroscope)
  add_noise/2(q_n) -> Controller/2(attitude)
  add_noise/3(v_n) -> Controller/3(velocity)
  add_noise/4(p_n) -> Controller/4(position)
  input/1 -> Controller/5(input)
  Controller/1(prop_speeds) -> Quadrotor/1(desired_propellor_speeds)

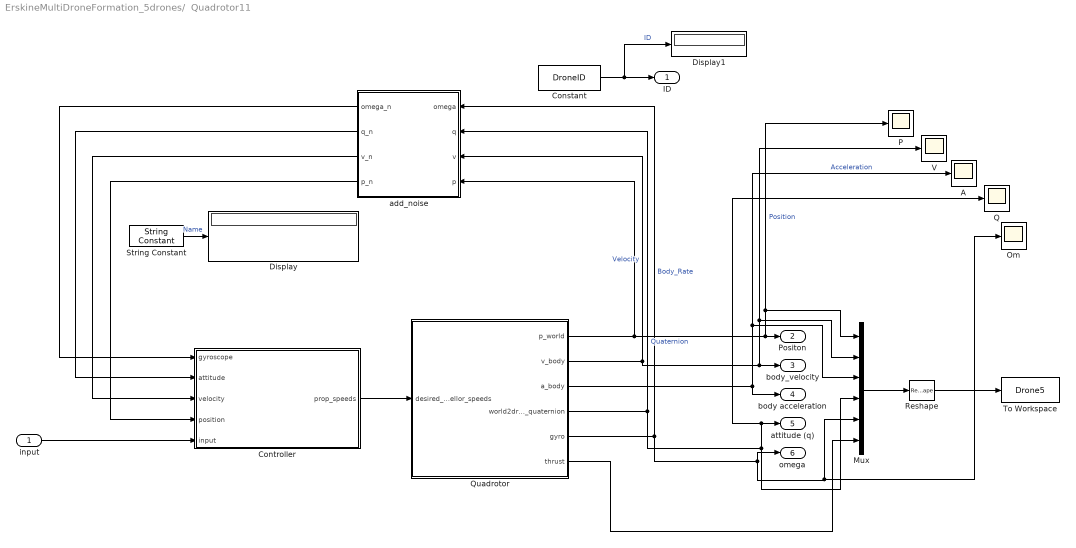
== system ErskineMultiDroneFormation_5drones/  Quadrotor11 ==
  input : Inport
  A : Scope
  Constant : Constant  Value=DroneID
  Controller : Subsystem
      mask Display: image('Format/flightController.png'); % Use "Edit Image" on toolstrip to change.
  Display : Display
  Display1 : Display
  Mux : Mux  Inputs=6
  Om : Scope
  P : Scope
  Q : Scope
  Quadrotor : Subsystem
      mask Display: image('droneHardware.jpeg'); % Use "Edit Image" on toolstrip to change.
  Reshape : Reshape
  String Constant : StringConstant  String=DroneName
  To Workspace : ToWorkspace  VariableName=Drone5  SaveFormat=Timeseries  SampleTime=-1
  V : Scope
  add_noise : MATLAB Function  TreatAsAtomicUnit=on
  ID : Outport
  Positon : Outport  Port=2
  body_velocity : Outport  Port=3
  body acceleration : Outport  Port=4
  attitude (q) : Outport  Port=5
  omega : Outport  Port=6
  wires:
  Quadrotor/5(gyro) -> Om/1, Mux/5, omega/1, add_noise/1(omega)  "Body_Rate"
  Quadrotor/1(p_world) -> add_noise/4(p), P/1, Mux/1, Positon/1  "Position"
  Quadrotor/3(a_body) -> body acceleration/1, A/1, Mux/3  "Acceleration"
  Quadrotor/4(world2drone_quaternion) -> Q/1, attitude (q)/1, Mux/4, add_noise/2(q)  "Quaternion"
  Mux/1 -> Reshape/1
  Quadrotor/2(v_body) -> V/1, Mux/2, body_velocity/1, add_noise/3(v)  "Velocity"
  Quadrotor/6(thrust) -> Mux/6
  String Constant/1 -> Display/1  "Name"
  Constant/1 -> Display1/1, ID/1  "ID"
  Reshape/1 -> To Workspace/1
  add_noise/1(omega_n) -> Controller/1(gyroscope)
  add_noise/2(q_n) -> Controller/2(attitude)
  add_noise/3(v_n) -> Controller/3(velocity)
  add_noise/4(p_n) -> Controller/4(position)
  input/1 -> Controller/5(input)
  Controller/1(prop_speeds) -> Quadrotor/1(desired_propellor_speeds)

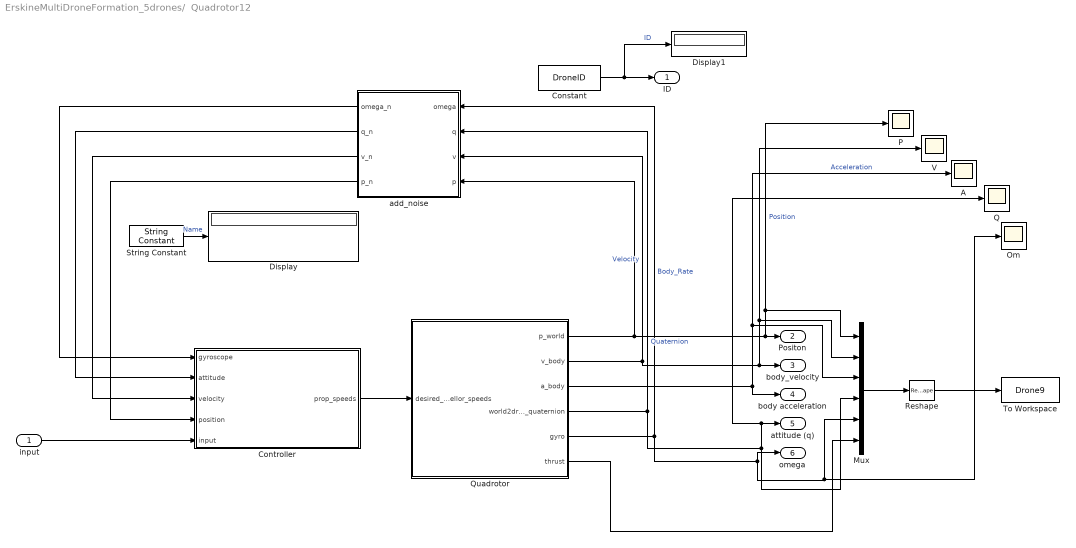
== system ErskineMultiDroneFormation_5drones/  Quadrotor12 ==
  input : Inport
  A : Scope
  Constant : Constant  Value=DroneID
  Controller : Subsystem
      mask Display: image('Format/flightController.png'); % Use "Edit Image" on toolstrip to change.
  Display : Display
  Display1 : Display
  Mux : Mux  Inputs=6
  Om : Scope
  P : Scope
  Q : Scope
  Quadrotor : Subsystem
      mask Display: image('droneHardware.jpeg'); % Use "Edit Image" on toolstrip to change.
  Reshape : Reshape
  String Constant : StringConstant  String=DroneName
  To Workspace : ToWorkspace  VariableName=Drone9  SaveFormat=Timeseries  SampleTime=-1
  V : Scope
  add_noise : MATLAB Function  TreatAsAtomicUnit=on
  ID : Outport
  Positon : Outport  Port=2
  body_velocity : Outport  Port=3
  body acceleration : Outport  Port=4
  attitude (q) : Outport  Port=5
  omega : Outport  Port=6
  wires:
  Quadrotor/5(gyro) -> Om/1, Mux/5, omega/1, add_noise/1(omega)  "Body_Rate"
  Quadrotor/1(p_world) -> add_noise/4(p), P/1, Mux/1, Positon/1  "Position"
  Quadrotor/3(a_body) -> body acceleration/1, A/1, Mux/3  "Acceleration"
  Quadrotor/4(world2drone_quaternion) -> Q/1, attitude (q)/1, Mux/4, add_noise/2(q)  "Quaternion"
  Mux/1 -> Reshape/1
  Quadrotor/2(v_body) -> V/1, Mux/2, body_velocity/1, add_noise/3(v)  "Velocity"
  Quadrotor/6(thrust) -> Mux/6
  String Constant/1 -> Display/1  "Name"
  Constant/1 -> Display1/1, ID/1  "ID"
  Reshape/1 -> To Workspace/1
  add_noise/1(omega_n) -> Controller/1(gyroscope)
  add_noise/2(q_n) -> Controller/2(attitude)
  add_noise/3(v_n) -> Controller/3(velocity)
  add_noise/4(p_n) -> Controller/4(position)
  input/1 -> Controller/5(input)
  Controller/1(prop_speeds) -> Quadrotor/1(desired_propellor_speeds)

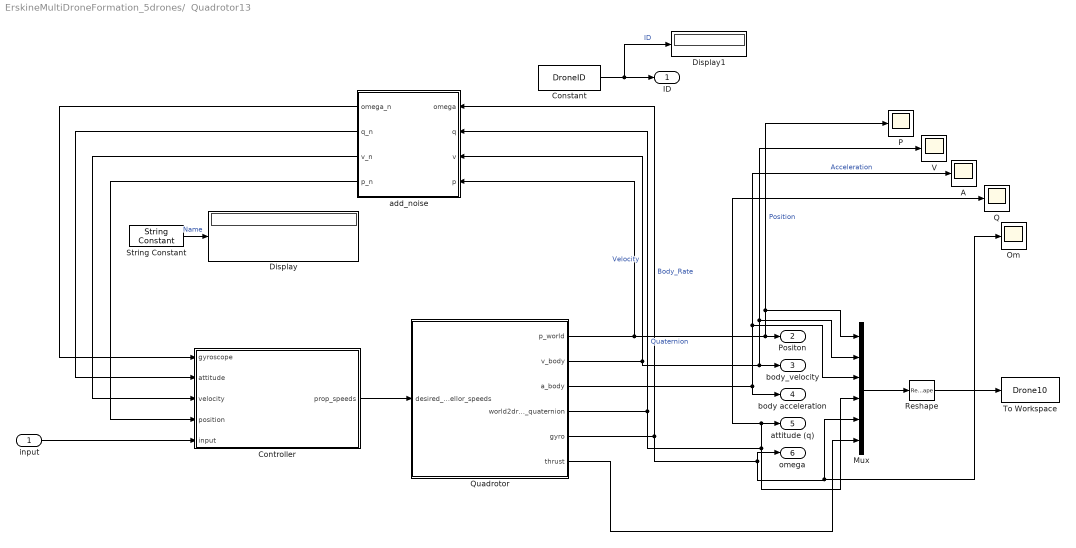
== system ErskineMultiDroneFormation_5drones/  Quadrotor13 ==
  input : Inport
  A : Scope
  Constant : Constant  Value=DroneID
  Controller : Subsystem
      mask Display: image('Format/flightController.png'); % Use "Edit Image" on toolstrip to change.
  Display : Display
  Display1 : Display
  Mux : Mux  Inputs=6
  Om : Scope
  P : Scope
  Q : Scope
  Quadrotor : Subsystem
      mask Display: image('droneHardware.jpeg'); % Use "Edit Image" on toolstrip to change.
  Reshape : Reshape
  String Constant : StringConstant  String=DroneName
  To Workspace : ToWorkspace  VariableName=Drone10  SaveFormat=Timeseries  SampleTime=-1
  V : Scope
  add_noise : MATLAB Function  TreatAsAtomicUnit=on
  ID : Outport
  Positon : Outport  Port=2
  body_velocity : Outport  Port=3
  body acceleration : Outport  Port=4
  attitude (q) : Outport  Port=5
  omega : Outport  Port=6
  wires:
  Quadrotor/5(gyro) -> Om/1, Mux/5, omega/1, add_noise/1(omega)  "Body_Rate"
  Quadrotor/1(p_world) -> add_noise/4(p), P/1, Mux/1, Positon/1  "Position"
  Quadrotor/3(a_body) -> body acceleration/1, A/1, Mux/3  "Acceleration"
  Quadrotor/4(world2drone_quaternion) -> Q/1, attitude (q)/1, Mux/4, add_noise/2(q)  "Quaternion"
  Mux/1 -> Reshape/1
  Quadrotor/2(v_body) -> V/1, Mux/2, body_velocity/1, add_noise/3(v)  "Velocity"
  Quadrotor/6(thrust) -> Mux/6
  String Constant/1 -> Display/1  "Name"
  Constant/1 -> Display1/1, ID/1  "ID"
  Reshape/1 -> To Workspace/1
  add_noise/1(omega_n) -> Controller/1(gyroscope)
  add_noise/2(q_n) -> Controller/2(attitude)
  add_noise/3(v_n) -> Controller/3(velocity)
  add_noise/4(p_n) -> Controller/4(position)
  input/1 -> Controller/5(input)
  Controller/1(prop_speeds) -> Quadrotor/1(desired_propellor_speeds)

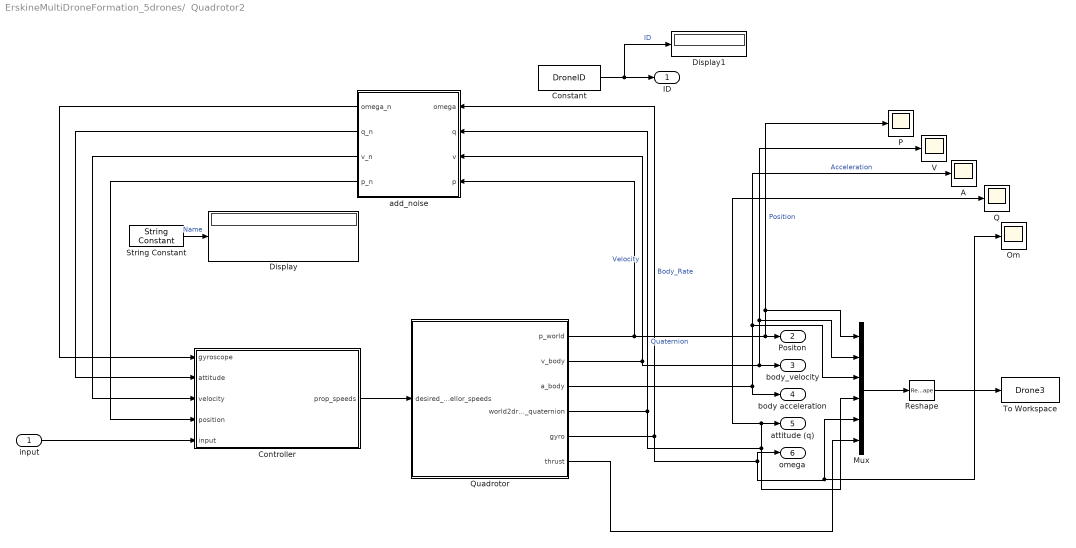
== system ErskineMultiDroneFormation_5drones/  Quadrotor2 ==
  input : Inport
  A : Scope
  Constant : Constant  Value=DroneID
  Controller : Subsystem
      mask Display: image('Format/flightController.png'); % Use "Edit Image" on toolstrip to change.
  Display : Display
  Display1 : Display
  Mux : Mux  Inputs=6
  Om : Scope
  P : Scope
  Q : Scope
  Quadrotor : Subsystem
      mask Display: image('droneHardware.jpeg'); % Use "Edit Image" on toolstrip to change.
  Reshape : Reshape
  String Constant : StringConstant  String=DroneName
  To Workspace : ToWorkspace  VariableName=Drone3  SaveFormat=Timeseries  SampleTime=-1
  V : Scope
  add_noise : MATLAB Function  TreatAsAtomicUnit=on
  ID : Outport
  Positon : Outport  Port=2
  body_velocity : Outport  Port=3
  body acceleration : Outport  Port=4
  attitude (q) : Outport  Port=5
  omega : Outport  Port=6
  wires:
  Quadrotor/5(gyro) -> Om/1, Mux/5, omega/1, add_noise/1(omega)  "Body_Rate"
  Quadrotor/1(p_world) -> add_noise/4(p), P/1, Mux/1, Positon/1  "Position"
  Quadrotor/3(a_body) -> body acceleration/1, A/1, Mux/3  "Acceleration"
  Quadrotor/4(world2drone_quaternion) -> Q/1, attitude (q)/1, Mux/4, add_noise/2(q)  "Quaternion"
  Mux/1 -> Reshape/1
  Quadrotor/2(v_body) -> V/1, Mux/2, body_velocity/1, add_noise/3(v)  "Velocity"
  Quadrotor/6(thrust) -> Mux/6
  String Constant/1 -> Display/1  "Name"
  Constant/1 -> Display1/1, ID/1  "ID"
  Reshape/1 -> To Workspace/1
  add_noise/1(omega_n) -> Controller/1(gyroscope)
  add_noise/2(q_n) -> Controller/2(attitude)
  add_noise/3(v_n) -> Controller/3(velocity)
  add_noise/4(p_n) -> Controller/4(position)
  input/1 -> Controller/5(input)
  Controller/1(prop_speeds) -> Quadrotor/1(desired_propellor_speeds)

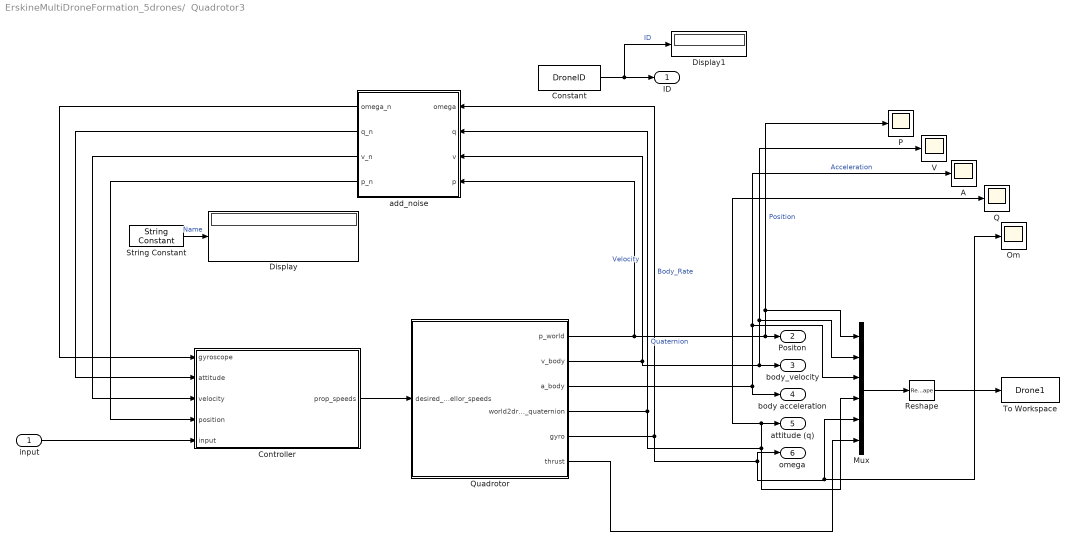
== system ErskineMultiDroneFormation_5drones/  Quadrotor3 ==
  input : Inport
  A : Scope
  Constant : Constant  Value=DroneID
  Controller : Subsystem
      mask Display: image('Format/flightController.png'); % Use "Edit Image" on toolstrip to change.
  Display : Display
  Display1 : Display
  Mux : Mux  Inputs=6
  Om : Scope
  P : Scope
  Q : Scope
  Quadrotor : Subsystem
      mask Display: image('droneHardware.jpeg'); % Use "Edit Image" on toolstrip to change.
  Reshape : Reshape
  String Constant : StringConstant  String=DroneName
  To Workspace : ToWorkspace  VariableName=Drone1  SaveFormat=Timeseries  SampleTime=-1
  V : Scope
  add_noise : MATLAB Function  TreatAsAtomicUnit=on
  ID : Outport
  Positon : Outport  Port=2
  body_velocity : Outport  Port=3
  body acceleration : Outport  Port=4
  attitude (q) : Outport  Port=5
  omega : Outport  Port=6
  wires:
  Quadrotor/5(gyro) -> Om/1, Mux/5, omega/1, add_noise/1(omega)  "Body_Rate"
  Quadrotor/1(p_world) -> add_noise/4(p), P/1, Mux/1, Positon/1  "Position"
  Quadrotor/3(a_body) -> body acceleration/1, A/1, Mux/3  "Acceleration"
  Quadrotor/4(world2drone_quaternion) -> Q/1, attitude (q)/1, Mux/4, add_noise/2(q)  "Quaternion"
  Mux/1 -> Reshape/1
  Quadrotor/2(v_body) -> V/1, Mux/2, body_velocity/1, add_noise/3(v)  "Velocity"
  Quadrotor/6(thrust) -> Mux/6
  String Constant/1 -> Display/1  "Name"
  Constant/1 -> Display1/1, ID/1  "ID"
  Reshape/1 -> To Workspace/1
  add_noise/1(omega_n) -> Controller/1(gyroscope)
  add_noise/2(q_n) -> Controller/2(attitude)
  add_noise/3(v_n) -> Controller/3(velocity)
  add_noise/4(p_n) -> Controller/4(position)
  input/1 -> Controller/5(input)
  Controller/1(prop_speeds) -> Quadrotor/1(desired_propellor_speeds)
